simulink model "IdentBuckSim2023b"  (R2023b)
settings: Solver=FixedStepAuto  StartTime=0.0  StopTime=1000*Tpwm  FixedStep=Tsim  RelTol=1e-3
values from neighbouring files (symbols this model uses):
  A = zeros(Ns-3,4)    [ident.m]    (also in identnew.m = [1,-1.99630021102880,0.996303145040676])
  B = [2.20050890435928e-05,4.40101780871856e-05,2.20050890435928e-05]    [identnew.m]
  Tpwm = 1/Fs    (= 0.001)    [ident.m]    (also in identnew.m)
  Tsim = Tpwm/100    (= 1e-05)    [ident.m]    (also in identnew.m)
  Vs = 30    [ident.m]    (also in identnew.m)
libraries: spsSeriesRLCBranchLib x3, spsDCVoltageSourceLib x1, spsDiodeLib x1, spsMosfetLib x1, commseqgen3 x1, simulink x1, spsVoltageMeasurementLib x1, sps_lib x1
settings Model: Creator=Raphael Teixeira  LastModifiedBy=luisf
settings RTWCC: GPUComputeCapability=5.0

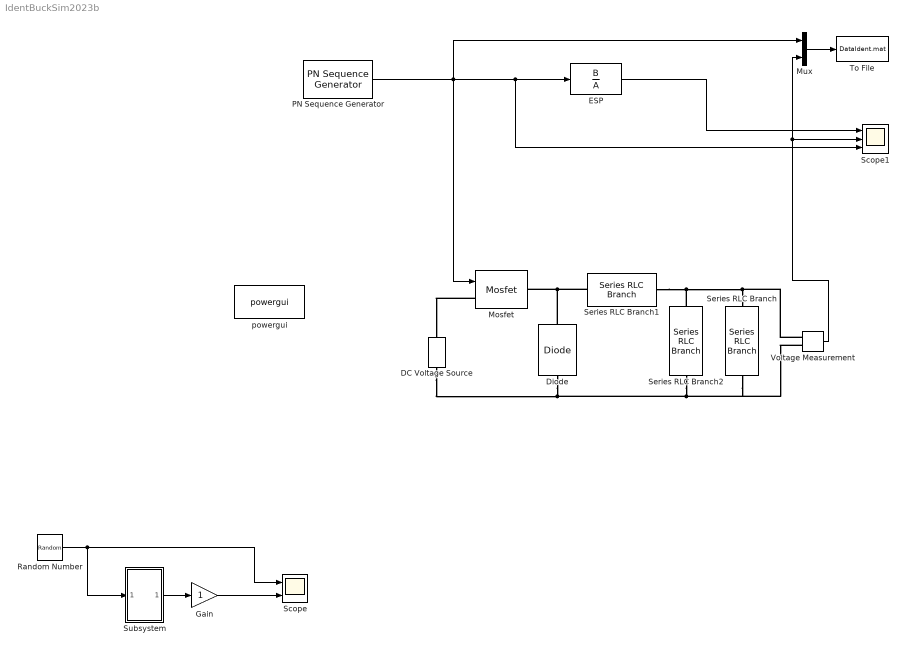
== system IdentBuckSim2023b ==
  DC Voltage Source : spsDCVoltageSourceLib/DC Voltage Source  Amplitude=Vs  Measurements=None
  Diode : spsDiodeLib/Diode  Ron=0.001  Lon=0  Vf=0.02  IC=0  UseSnubber=0  Rs=500  Cs=250e-9  Measurements=off
  ESP : DiscreteTransferFcn  Numerator=B  Denominator=A
  Gain : Gain  OutDataTypeStr=double
  Mosfet : spsMosfetLib/Mosfet  Ron=0.01  Lon=0  Rd=0.01  Vfd=0  IC=0  Rs=1e5  Cs=inf  Measurements=off
  Mux : Mux  Inputs=2
  PN Sequence Generator : commseqgen3/PN Sequence Generator  poly=[15 14 0]  ini_sta=ones(1, 15)  outBitMaskSource=Dialog parameter  shift=0  outVarSiz=off  maxOutSizeMode=Dialog parameter  maxOutSize=[10 1]  Ts=Tsim  sampPerFrame=1  reset=off  bitPackedOutputs=off  outDataType=double  numPackedBits=8  bitPackDataSigned=off  bitPackedOutDType=double
  Random Number : RandomNumber  Mean=15  Variance=5  SampleTime=Tpwm
  Scope : Scope  NumInputPorts=2
  Scope1 : Scope  NumInputPorts=3
  Series RLC Branch : spsSeriesRLCBranchLib/Series RLC Branch  LConnTagsString=__new0  RConnTagsString=__new0  BranchType=R  Resistance=1  Inductance=1e-3  SetiL0=off  InitialCurrent=0  Capacitance=1e-6  Setx0=off  InitialVoltage=0  Measurements=None
  Series RLC Branch1 : spsSeriesRLCBranchLib/Series RLC Branch  LConnTagsString=__new0  RConnTagsString=__new0  BranchType=L  Resistance=1  Inductance=0.0126  SetiL0=off  InitialCurrent=0  Capacitance=1e-6  Setx0=off  InitialVoltage=0  Measurements=None
  Series RLC Branch2 : spsSeriesRLCBranchLib/Series RLC Branch  LConnTagsString=__new0  RConnTagsString=__new0  BranchType=C  Resistance=1  Inductance=1e-3  SetiL0=off  InitialCurrent=0  Capacitance=0.0027  Setx0=off  InitialVoltage=0  Measurements=None
  Subsystem : Subsystem
  To File : ToFile  Filename=DataIdent.mat  MatrixName=DadosBuck
  Voltage Measurement : spsVoltageMeasurementLib/Voltage Measurement  PhasorSimulation=off  OutputType=Complex  PSBequivalent=0
  powergui : sps_lib/powergui  Priority=1  SimulationMode=Continuous  SampleTime=50e-6  frequency=60  Iterations=50  frequencyindice=0  Pbase=100e6  ErrMax=1e-4  UnitsV=kV  UnitsW=MW  buscounter=0  FunctionMessages=off  echomessages=off  EnableUseOfTLC=off  CurrentSourceSwitches=off  DisableSnubberDevices=off  DisableRonSwitches=off  DisableVfSwitches=off  DisplayEquations=off  AutomaticDiscreteSolvers=off  SolverType=Tustin/Backward Euler (TBE)  Interpol=off  ExternalGateDelay=off  methode=off  Ts=100  x0status=blocks  SPID=on  SwTol=0  HookPort=off  NonlinearTolerance=1e-4  nMaxIteration=100  ContinueOnMaxIteration=off  RestoreLinks=warning  ResistiveCurrentMeasurement=off  Frange=[0:2:500]  Ylog=off  Xlog=on  ShowGrid=off  save=off  variable=ZData  structure=0  ZoomFFT=off  StartTime=0.0  cycles=1  DisplayStyle=1  fundamental=60  FreqAxis=off  MaxFrequency=1000  frequencyindicesteady=1  RmsSteady=1  display=off
  wires:
  Random Number/1 -> Scope/1, Subsystem/1(In1)
  Voltage Measurement/1 -> Mux/2, Scope1/2
  Mux/1 -> To File/1
  Subsystem/1(Out1) -> Gain/1
  Gain/1 -> Scope/2
  ESP/1 -> Scope1/1
  PN Sequence Generator/1 -> Mosfet/1, Mux/1, Scope1/3, ESP/1
  connections:
  Series RLC Branch2/LConn1 -- Series RLC Branch/LConn1 -- Voltage Measurement/LConn1 -- Series RLC Branch1/RConn1
  Diode/LConn1 -- DC Voltage Source/LConn1 -- Series RLC Branch/RConn1 -- Voltage Measurement/LConn2 -- Series RLC Branch2/RConn1
  Diode/RConn1 -- Mosfet/RConn1 -- Series RLC Branch1/LConn1
  Mosfet/LConn1 -- DC Voltage Source/RConn1

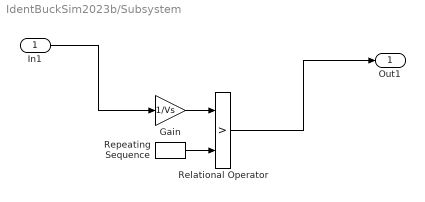
== system IdentBuckSim2023b/Subsystem ==
  In1 : Inport
  Gain : Gain  Gain=1/Vs
  Relational Operator : RelationalOperator  Operator=>  OutDataTypeStr=boolean  RndMeth=Simplest  InputSameDT=off
  Repeating Sequence : simulink/Sources/Repeating Sequence  rep_seq_t=[0 Tpwm]  rep_seq_y=[0 1]
  Out1 : Outport
  wires:
  Relational Operator/1 -> Out1/1
  Repeating Sequence/1 -> Relational Operator/2
  Gain/1 -> Relational Operator/1
  In1/1 -> Gain/1
